simulink model "autosar_multirunnables_top_PIL"  (R2018b)
settings: Solver=FixedStepDiscrete  StartTime=0.0  StopTime=200  FixedStep=0.1  RelTol=1e-3  EnableMultiTasking=on
InitFcn:
  | mbd_s32k_as_consistency_checks(bdroot(gcs));
undefined symbols (not defined in the file): sigbuilder_block
libraries: simulink x3
Description:
  | This model shows how to run an AUTOSAR Multi Runnable simulation in PIL mode on S32K targets.
  | The model is based on the Matlab's AUTOSAR Blockset Toolbox example.
  | For more details please follow the link https://www.mathworks.com/videos/autosar-code-generation-for-multiple-runnable-entities-102137.html
  | 
  | In order to run this model in PIL simulation on target, the following steps must be followed:
  | 1. Open the reference 'autosar_integrator_PIL' model.
  | 2. Open the 'MBD_S32K1xx_AUTOSAR_Config_Information' block. If you want to run a custom/another AUTOSAR compliant model in PIL, once it runs in simulation as expected, this block must be added in the model.
  | It will change the System target file and will perform the model settings for code build and target deployment.
  | 3. In the MCU Tab chose the processor on which you want to run the model. For S32K11x EVB, the Clock and XTAL Frequency must be 40 MHz/External 40MHz. For the other boards the frequencies must be chosen
  | 80/External 8 MHz.
  | 4. In Build Toolchain Tab select the Compiler which you want to use.
  | 5. In Target Connection Tab Select the Download Interface type: Serial/OpenSDA. The Serial Group selects the computer COM port on which the Matlab model will exchange data with the target and the desired Baud Rate.
  | The OpenSDA group will be active only if the Download Interface is OpenSDA. Here, the right EVB Drive Name must be selected.
  | The PIL Settings Tab selects the EVB board LPUART instance and pins used for the PIL Serial communication. For the S32K11x must be selected the LPUART0/PTB0/PTB1 configuration. For the S32K14x must be selected
  | the LPUART1/PTC6/PTC7 configuration.
  | 6. Save the model and return to the top model.
  | 7. If the top model was never been run on the S32K board, go tho Tools>NXP Model-Based Design AUTOSAR Toolbox for  S32K1xx MCUs>To PIL Mode on S32K.
  | 8. Press Run button.
  | The code will be generated, compiledd, deployed and run on the target.
settings Model: Creator=NXP MBDT Team  LastModifiedBy=shivama
settings DataIOCC: ExternalInput=off  InitialState=off  SaveFormat=Array  SignalLoggingSaveFormat=ModelDataLogs  SaveOutput=off  SignalLogging=off  SaveTime=off
settings OptimizationCC: DefaultParameterBehavior=Inlined  UseDivisionForNetSlopeComputation=on  EnhancedBackFolding=on  PassReuseOutputArgsAs=Individual arguments  ExpressionDepthLimit=2147483647  ZeroExternalMemoryAtStartup=off  ZeroInternalMemoryAtStartup=off  OptimizeBlockOrder=speed  DifferentSizesBufferReuse=on
settings DebuggingCC: SolverPrmCheckMsg=warning  InheritedTsInSrcMsg=none  SingleTaskRateTransMsg=error  ParameterTunabilityLossMsg=error  FcnCallInpInsideContextMsg=warning  UnconnectedInputMsg=error  UnconnectedOutputMsg=error  UnconnectedLineMsg=error  UnknownTsInhSupMsg=error  StateNameClashWarn=warning  SFUnexpectedBacktrackingDiag=warning  SFNoUnconditionalDefaultTransitionDiag=warning  SFExecutionAtInitializationDiag=none
settings HardwareCC: ProdBitPerPointer=32  ProdBitPerSizeT=32  ProdBitPerPtrDiffT=32  ProdLargestAtomicInteger=Long  ProdLargestAtomicFloat=Double  ProdWordSize=32  ProdHWDeviceType=ARM Compatible->ARM Cortex
settings ModelReferenceCC: UpdateModelReferenceTargets=Force  PropagateSignalLabelsOutOfModel=off
settings SFSimCC: SimUseLocalCustomCode=off  MATLABDynamicMemAlloc=off
settings RTWCC: SystemTargetFile=mbd_s32k_as.tlc  MakeCommand=mbd_s32k_as_make_rtw COPY_MDLREF_INCLUDES=0  TemplateMakefile=mbd_s32k_as.tmf  PostCodeGenCommand=mcd_567xf_analyzegencode(buildInfo)  Description=Model Based Design Autosar Toolbox S32K Code Generation Target  GenerateReport=on  RTWUseLocalCustomCode=off  IncludeHyperlinkInReport=on  LaunchReport=on  CodeExecutionProfiling=on  CodeProfilingSaveOptions=AllData  CodeProfilingInstrumentation=detailed  GenerateTraceInfo=on  GenerateTraceReport=on  GenerateTraceReportSl=on  GenerateTraceReportSf=on  GenerateTraceReportEml=on
settings CodeAppCC: ForceParamTrailComments=on  IgnoreCustomStorageClasses=off  MaxIdLength=63  OperatorAnnotations=on  SimulinkDataObjDesc=on  SFDataObjDesc=on  InsertBlockDesc=on
settings STFCustomTargetCC: MultiwordLength=256  ParMdlRefBuildCompliant=on  CompOptLevelCompliant=on  IncludeMdlTerminateFcn=off  CombineOutputUpdateFcns=on  SuppressErrorStatus=on  ERTCustomFileBanners=on  SupportAbsoluteTime=off  SupportNonFinite=off  SupportComplex=off  SupportContinuousTime=off  SupportNonInlinedSFcns=off  RemoveResetFunc=on  MATLABClassNameForMDSCustomization=Simulink.SoftwareTarget.ERTCustomization  AutosarCompliant=on  LookupTableObjectStructAxisOrder=2,1,3,4,...  LUTObjectStructOrderEvenSpacing=Size,Table,Breakpoints  SystemTargetFile=mbd_s32k_as.tlc
settings ERTTargetCC: ConcurrentExecutionCompliant=off  IncludeMdlTerminateFcn=off  SuppressErrorStatus=on  SupportAbsoluteTime=off  SupportNonFinite=off  SupportComplex=off  ModelStepFunctionPrototypeControlCompliant=off  CPPClassGenCompliant=off  AutosarCompliant=on  UseToolchainInfoCompliant=off  LookupTableObjectStructAxisOrder=2,1,3,4,...  LUTObjectStructOrderEvenSpacing=Size,Table,Breakpoints  InlinedParameterPlacement=NonHierarchical  ERTCustomFileTemplate=example_file_process.tlc
settings ConfigComp: CovMetricSettings=dw  CovHtmlReporting=on  CovSaveCumulativeToWorkspaceVar=on  CovSaveSingleToWorkspaceVar=on  CovExternalEMLEnable=off

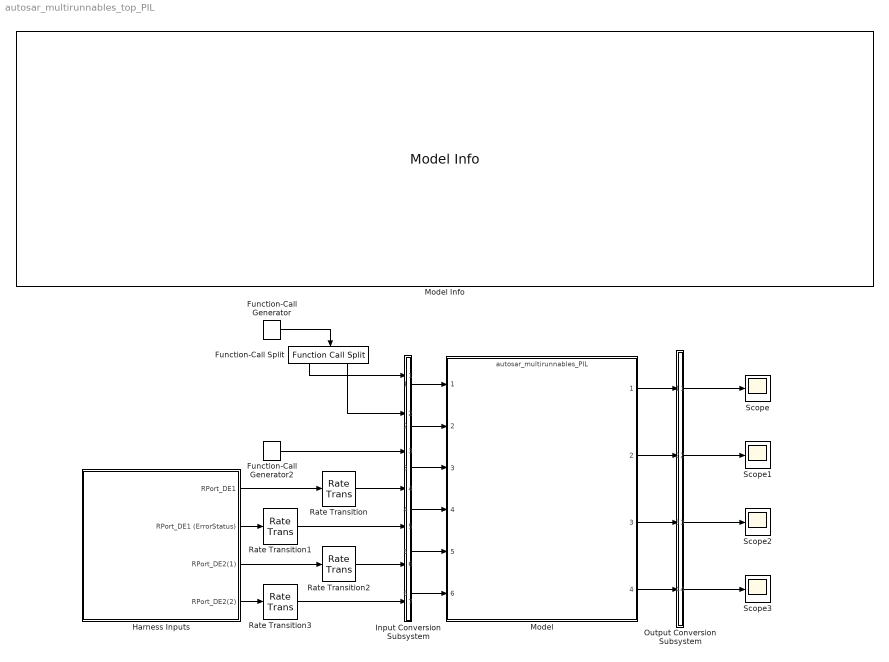
== system autosar_multirunnables_top_PIL ==
  Function-Call Generator : simulink/Ports & Subsystems/Function-Call Generator  sample_time=1  numberOfIterations=1
  Function-Call Generator2 : simulink/Ports & Subsystems/Function-Call Generator  sample_time=10  numberOfIterations=1
  Function-Call Split : FunctionCallSplit  IconShape=distinctive  NumOutputPorts=2
  Harness Inputs : Subsystem  Tag=STV Subsys  LoadFcn=sigbuilder_block('load');  StartFcn=sigbuilder_block('start');  StopFcn=sigbuilder_block('stop');  ClipboardFcn=sigbuilder_block('clipboard');  mask(Sigbuilder block){tuvar=[0:10]}
      mask init:
      | if ~strcmp(get_param(bdroot(gcb),'SimulationStatus'),'stopped'),tuvar = sigbuilder_block('maskInit'); end
      settings: CopyFcn=sigbuilder_block('copy');  DeleteFcn=sigbuilder_block('delete');  ModelCloseFcn=sigbuilder_block('modelClose');  PreSaveFcn=sigbuilder_block('preSave');  PauseFcn=sigbuilder_block('pause');  ContinueFcn=sigbuilder_block('continue');  NameChangeFcn=sigbuilder_block('namechange');  OpenFcn=sigbuilder_block('open',[50 50 520 400 ]);  CloseFcn=sigbuilder_block('close');
      mask Display: plot(0, 0, 100, 100,[2, 2, 32, 32, 2], [68, 8, 8, 68, 68],[32, 2], [38, 38], [32, 19, 2],[53, 60, 44], [32, 17, 17, 2],[16, 16, 31, 31]);txt = getActiveGroup(gcbh);text(2, 100, txt,'verticalAlignment', 'top');
  Input Conversion Subsystem : Subsystem  Tag=_input_conv_ss_
  Model : ModelReference  ModelNameDialog=autosar_multirunnables_PIL.slx  SimulationMode=Processor-in-the-loop (PIL)  ShowModelPeriodicEventPorts=on  CodeInterface=Top model  ModelReferenceVersion=1.383
  Model Info : simulink/Model-Wide Utilities/Model Info  Frame=off  DisplayStringWithTags=|  HorizontalTextAlignment=Left  LeftAlignmentValue=0.02
      | Model Name: %<ModelName>
      | 
      | Description: %<Description>
  Output Conversion Subsystem : Subsystem  Tag=_output_conv_ss_
  Rate Transition{,1..3} (4 alike) : RateTransition
  Scope{,1..3} (4 alike) : Scope
  wires:
  Input Conversion Subsystem/1(Out_1) -> Model/1
  Input Conversion Subsystem/2(Out_2) -> Model/2
  Input Conversion Subsystem/3(Out_3) -> Model/3
  Input Conversion Subsystem/4(Out_4) -> Model/4
  Input Conversion Subsystem/5(Out_5) -> Model/5
  Input Conversion Subsystem/6(Out_6) -> Model/6
  Function-Call Generator/1 -> Function-Call Split/1
  Function-Call Generator2/1 -> Input Conversion Subsystem/3(In_3)
  Model/1 -> Output Conversion Subsystem/1(In_1)
  Model/2 -> Output Conversion Subsystem/2(In_2)
  Model/3 -> Output Conversion Subsystem/3(In_3)
  Model/4 -> Output Conversion Subsystem/4(In_4)
  Output Conversion Subsystem/2(Out_2) -> Scope1/1
  Output Conversion Subsystem/3(Out_3) -> Scope2/1
  Output Conversion Subsystem/1(Out_1) -> Scope/1
  Output Conversion Subsystem/4(Out_4) -> Scope3/1
  Harness Inputs/1(RPort_DE1) -> Rate Transition/1
  Harness Inputs/2(RPort_DE1 (ErrorStatus)) -> Rate Transition1/1
  Harness Inputs/3(RPort_DE2(1)) -> Rate Transition2/1
  Harness Inputs/4(RPort_DE2(2)) -> Rate Transition3/1
  Rate Transition/1 -> Input Conversion Subsystem/4(In_4)
  Rate Transition1/1 -> Input Conversion Subsystem/5(In_5)
  Rate Transition2/1 -> Input Conversion Subsystem/6(In_6)
  Rate Transition3/1 -> Input Conversion Subsystem/7(In_7)
  Function-Call Split/1 -> Input Conversion Subsystem/1(In_1)
  Function-Call Split/2 -> Input Conversion Subsystem/2(In_2)

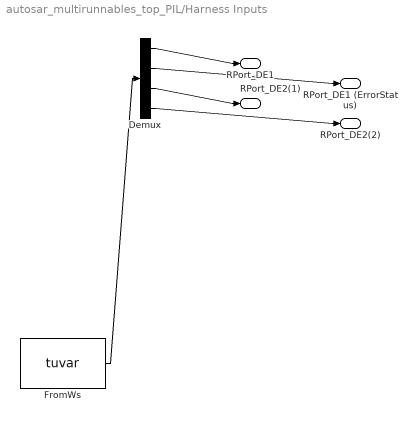
== system autosar_multirunnables_top_PIL/Harness Inputs ==
  Demux : Demux  Tag=STV Demux
  FromWs : FromWorkspace  Tag=STV FromWs  VariableName=tuvar  SampleTime=0
      SigBuilderData=|
      | dataSet.timeRange = [0 1]
      | dataSet.name = 'Group 1'
      | sbobj.Name = 'Signal Builder'
      | sbobj.Groups.Name = 'Group 1'
      | sbobj.Groups.Signals(1).Name = 'RPort_DE1'
      | sbobj.Groups.Signals(1).XData = [0 1]
      | sbobj.Groups.Signals(1).YData = [1 1]
      | sbobj.Groups.Signals(2).Name = 'RPort_DE1 (ErrorStatus)'
      | sbobj.Groups.Signals(2).XData = [0 1]
      | sbobj.Groups.Signals(2).YData = [1 1]
      | sbobj.Groups.Signals(3).Name = 'RPort_DE2(1)'
      | sbobj.Groups.Signals(3).XData = [0 1]
      | sbobj.Groups.Signals(3).YData = [1 1]
      | sbobj.Groups.Signals(4).Name = 'RPort_DE2(2)'
      | sbobj.Groups.Signals(4).XData = [0 1]
      | sbobj.Groups.Signals(4).YData = [1 1]
      | sbobj.Groups.TimeRange = [0 1]
  RPort_DE1 : Outport  Tag=STV Outport
  RPort_DE1 (ErrorStatus) : Outport  Tag=STV Outport  Port=2
  RPort_DE2(1) : Outport  Tag=STV Outport  Port=3
  RPort_DE2(2) : Outport  Tag=STV Outport  Port=4
  wires:
  FromWs/1 -> Demux/1
  Demux/1 -> RPort_DE1/1
  Demux/2 -> RPort_DE1 (ErrorStatus)/1
  Demux/3 -> RPort_DE2(1)/1
  Demux/4 -> RPort_DE2(2)/1

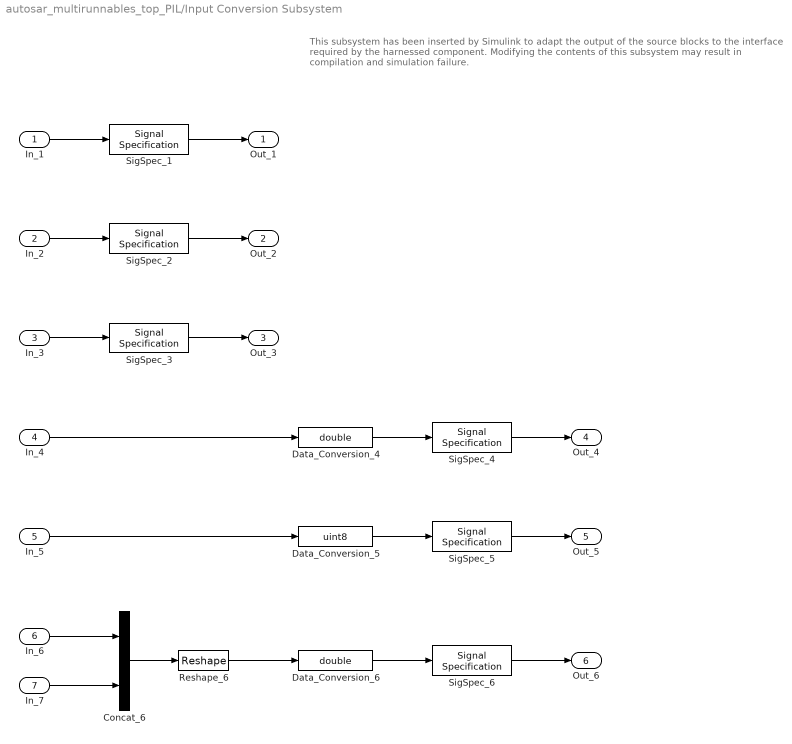
== system autosar_multirunnables_top_PIL/Input Conversion Subsystem ==
  note: This subsystem has been inserted by Simulink to adapt the output of the source blocks to the interface required by the harnessed component.
      |  Modifying the contents of this subsystem may result in compilation and simulation failure.
  In_1 : Inport
  In_2 : Inport  Port=2
  In_3 : Inport  Port=3
  In_4 : Inport  Port=4
  In_5 : Inport  Port=5
  In_6 : Inport  Port=6
  In_7 : Inport  Port=7
  Concat_6 : Concatenate
  Data_Conversion_4 : DataTypeConversion  OutDataTypeStr=double  SaturateOnIntegerOverflow=on  RndMeth=Zero
  Data_Conversion_5 : DataTypeConversion  OutDataTypeStr=uint8  SaturateOnIntegerOverflow=on  RndMeth=Zero
  Data_Conversion_6 : DataTypeConversion  OutDataTypeStr=double  SaturateOnIntegerOverflow=on  RndMeth=Zero
  Reshape_6 : Reshape  OutputDimensionality=Customize  OutputDimensions=[2]
  SigSpec_1 : SignalSpecification
  SigSpec_2 : SignalSpecification
  SigSpec_3 : SignalSpecification
  SigSpec_4 : SignalSpecification  OutDataTypeStr=double  Dimensions=[1]  SampleTime=[-1 0]
  SigSpec_5 : SignalSpecification  OutDataTypeStr=uint8  Dimensions=[1]  SampleTime=[-1 0]
  SigSpec_6 : SignalSpecification  OutDataTypeStr=double  Dimensions=[2]  SampleTime=[-1 0]
  Out_1 : Outport
  Out_2 : Outport  Port=2
  Out_3 : Outport  Port=3
  Out_4 : Outport  Port=4
  Out_5 : Outport  Port=5
  Out_6 : Outport  Port=6
  wires:
  In_6/1 -> Concat_6/1
  In_7/1 -> Concat_6/2
  Concat_6/1 -> Reshape_6/1
  In_4/1 -> Data_Conversion_4/1
  In_5/1 -> Data_Conversion_5/1
  Reshape_6/1 -> Data_Conversion_6/1
  In_1/1 -> SigSpec_1/1
  In_2/1 -> SigSpec_2/1
  In_3/1 -> SigSpec_3/1
  Data_Conversion_4/1 -> SigSpec_4/1
  Data_Conversion_5/1 -> SigSpec_5/1
  Data_Conversion_6/1 -> SigSpec_6/1
  SigSpec_1/1 -> Out_1/1
  SigSpec_2/1 -> Out_2/1
  SigSpec_3/1 -> Out_3/1
  SigSpec_4/1 -> Out_4/1
  SigSpec_5/1 -> Out_5/1
  SigSpec_6/1 -> Out_6/1

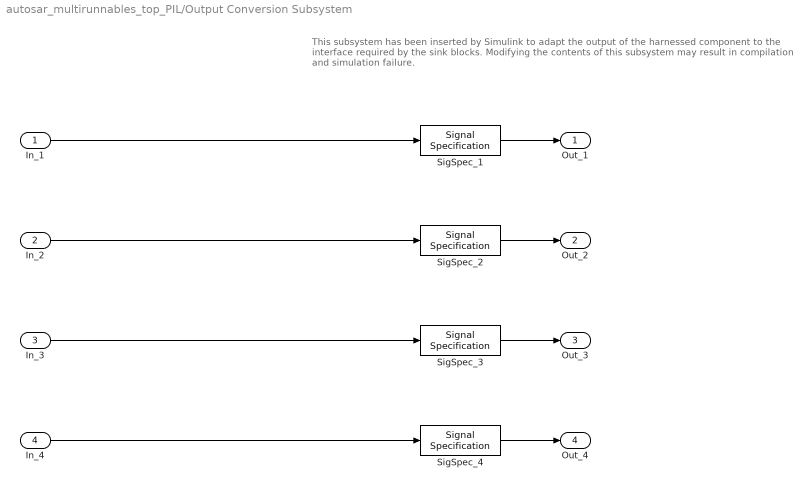
== system autosar_multirunnables_top_PIL/Output Conversion Subsystem ==
  note: This subsystem has been inserted by Simulink to adapt the output of the harnessed component to the interface required by the sink blocks.
      |  Modifying the contents of this subsystem may result in compilation and simulation failure.
  In_1 : Inport
  In_2 : Inport  Port=2
  In_3 : Inport  Port=3
  In_4 : Inport  Port=4
  SigSpec_1 : SignalSpecification  OutDataTypeStr=int8  Dimensions=[1]
  SigSpec_2 : SignalSpecification  OutDataTypeStr=int8  Dimensions=[1]
  SigSpec_3 : SignalSpecification  OutDataTypeStr=int8  Dimensions=[2]
  SigSpec_4 : SignalSpecification  OutDataTypeStr=double  Dimensions=[1]
  Out_1 : Outport
  Out_2 : Outport  Port=2
  Out_3 : Outport  Port=3
  Out_4 : Outport  Port=4
  wires:
  SigSpec_1/1 -> Out_1/1
  SigSpec_2/1 -> Out_2/1
  SigSpec_3/1 -> Out_3/1
  SigSpec_4/1 -> Out_4/1
  In_1/1 -> SigSpec_1/1
  In_2/1 -> SigSpec_2/1
  In_3/1 -> SigSpec_3/1
  In_4/1 -> SigSpec_4/1
